simulink model "RiceCooker"  (R2023b)
settings: Solver=FixedStepAuto  StartTime=0.0  StopTime=10*60  RelTol=1e-3
undefined symbols (not defined in the file): m_0, T_0
settings Model: Creator=20181234  LastModifiedBy=20181234

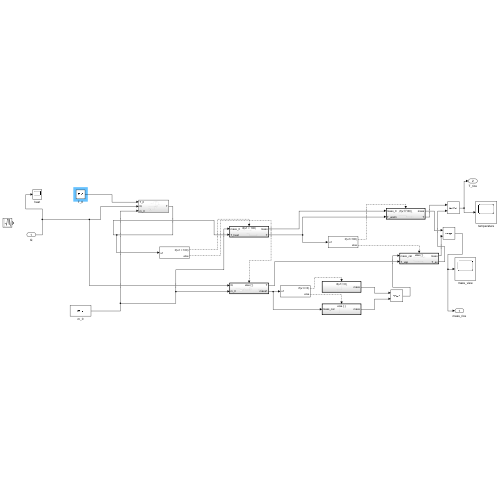
[thumbnail: Simulink's stored preview of the top-level diagram]
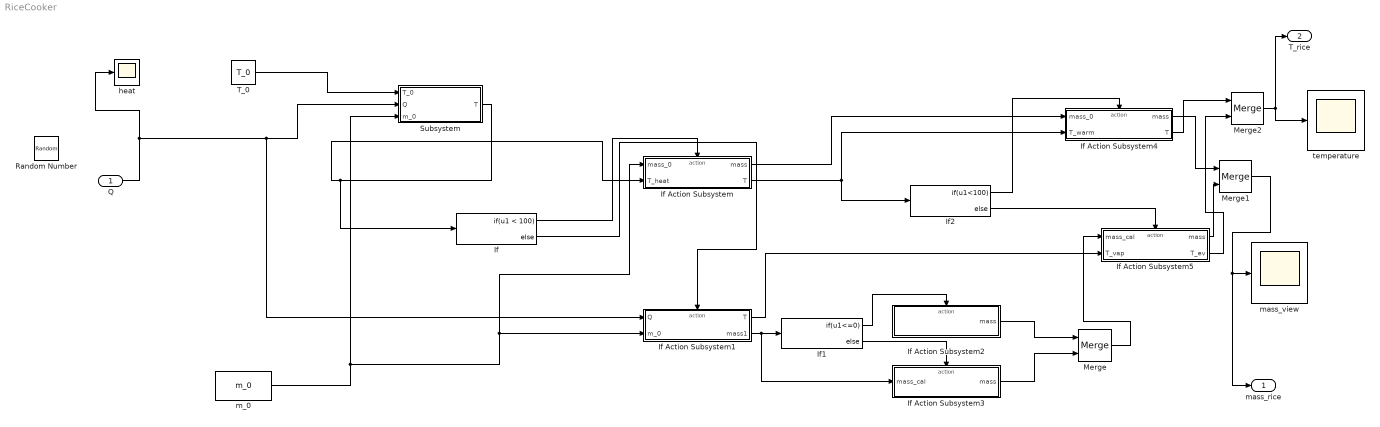
== system RiceCooker ==
  Q : Inport
  If : If  IfExpression=u1 < 100
  If Action Subsystem : Subsystem  TreatAsAtomicUnit=on
  If Action Subsystem1 : Subsystem  TreatAsAtomicUnit=on
  If Action Subsystem2 : Subsystem  TreatAsAtomicUnit=on
  If Action Subsystem3 : Subsystem  TreatAsAtomicUnit=on
  If Action Subsystem4 : Subsystem  TreatAsAtomicUnit=on
  If Action Subsystem5 : Subsystem  TreatAsAtomicUnit=on
  If1 : If  IfExpression=u1<=0
  If2 : If  IfExpression=u1<100
  Merge : Merge
  Merge1 : Merge
  Merge2 : Merge
  Random Number : RandomNumber  Mean=4500  Variance=500  Seed=65981  SampleTime=0.5
  Subsystem : Subsystem
  T_0 : Constant  Value=T_0
  heat : Scope
  m_0 : Constant  Value=m_0
  mass_view : Scope
  temperature : Scope
  mass_rice : Outport
  T_rice : Outport  Port=2
  wires:
  T_0/1 -> Subsystem/1(T_0)
  Q/1 -> heat/1, If Action Subsystem1/1(Q), Subsystem/2(Q)
  m_0/1 -> If Action Subsystem1/2(m_0), If Action Subsystem/1(mass_0), Subsystem/3(m_0)
  Subsystem/1(T) -> If/1, If Action Subsystem/2(T_heat)
  If/1 -> If Action Subsystem/Action
  If/2 -> If Action Subsystem1/Action
  If Action Subsystem/2(T) -> If Action Subsystem4/2(T_warm), If2/1
  If Action Subsystem1/2(mass1) -> If Action Subsystem3/1(mass_cal), If1/1
  If1/1 -> If Action Subsystem2/Action
  If1/2 -> If Action Subsystem3/Action
  If Action Subsystem2/1(mass) -> Merge/1
  If Action Subsystem3/1(mass) -> Merge/2
  Merge/1 -> If Action Subsystem5/1(mass_cal)
  If2/2 -> If Action Subsystem5/Action
  If2/1 -> If Action Subsystem4/Action
  If Action Subsystem4/1(mass) -> Merge1/1
  If Action Subsystem5/1(mass) -> Merge1/2
  Merge1/1 -> mass_rice/1, mass_view/1
  If Action Subsystem/1(mass) -> If Action Subsystem4/1(mass_0)
  If Action Subsystem4/2(T) -> Merge2/1
  If Action Subsystem5/2(T_ev) -> Merge2/2
  Merge2/1 -> T_rice/1, temperature/1
  If Action Subsystem1/1(T) -> If Action Subsystem5/2(T_vap)

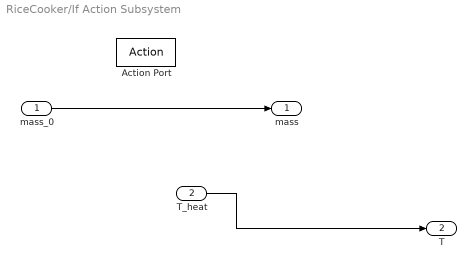
== system RiceCooker/If Action Subsystem ==
  mass_0 : Inport
  T_heat : Inport  Port=2
  Action Port : ActionPort  ActionPortLabel=if(u1 < 100)
  mass : Outport
  T : Outport  Port=2
  wires:
  mass_0/1 -> mass/1
  T_heat/1 -> T/1

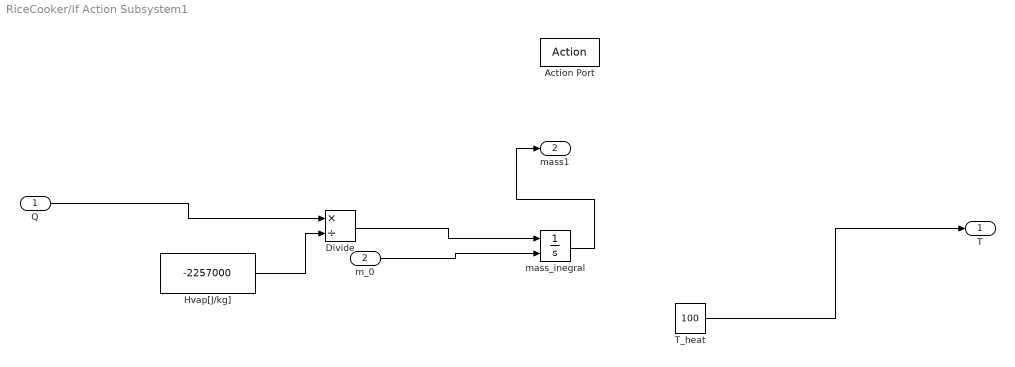
== system RiceCooker/If Action Subsystem1 ==
  Q : Inport
  m_0 : Inport  Port=2
  Action Port : ActionPort  ActionPortLabel=else
  Divide : Product  Inputs=*/
  Hvap[J/kg] : Constant  Value=-2257000
  T_heat : Constant  Value=100
  mass_inegral : Integrator  InitialConditionSource=external
  T : Outport
  mass1 : Outport  Port=2
  wires:
  Hvap[J/kg]/1 -> Divide/2
  m_0/1 -> mass_inegral/2
  mass_inegral/1 -> mass1/1
  Q/1 -> Divide/1
  Divide/1 -> mass_inegral/1
  T_heat/1 -> T/1

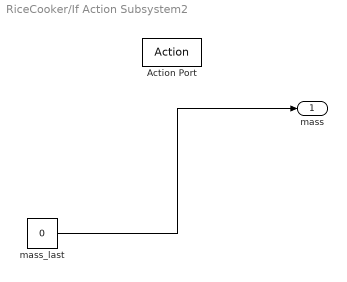
== system RiceCooker/If Action Subsystem2 ==
  Action Port : ActionPort  ActionPortLabel=if(u1<=0)
  mass_last : Constant  Value=0
  mass : Outport
  wires:
  mass_last/1 -> mass/1

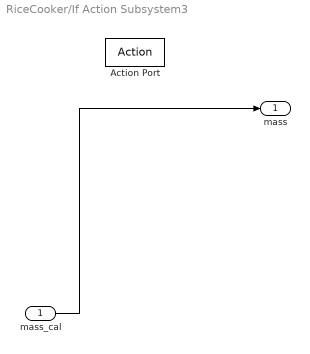
== system RiceCooker/If Action Subsystem3 ==
  mass_cal : Inport
  Action Port : ActionPort  ActionPortLabel=else
  mass : Outport
  wires:
  mass_cal/1 -> mass/1

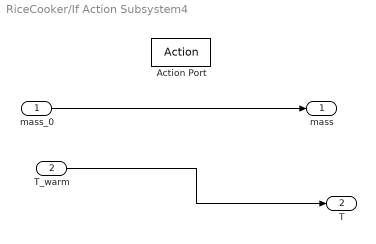
== system RiceCooker/If Action Subsystem4 ==
  mass_0 : Inport
  T_warm : Inport  Port=2
  Action Port : ActionPort  ActionPortLabel=if(u1<100)
  mass : Outport
  T : Outport  Port=2
  wires:
  mass_0/1 -> mass/1
  T_warm/1 -> T/1

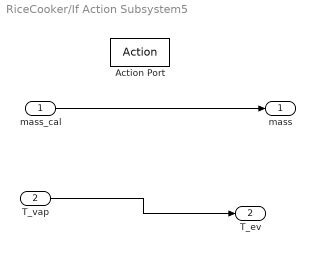
== system RiceCooker/If Action Subsystem5 ==
  mass_cal : Inport
  T_vap : Inport  Port=2
  Action Port : ActionPort  ActionPortLabel=else
  mass : Outport
  T_ev : Outport  Port=2
  wires:
  mass_cal/1 -> mass/1
  T_vap/1 -> T_ev/1

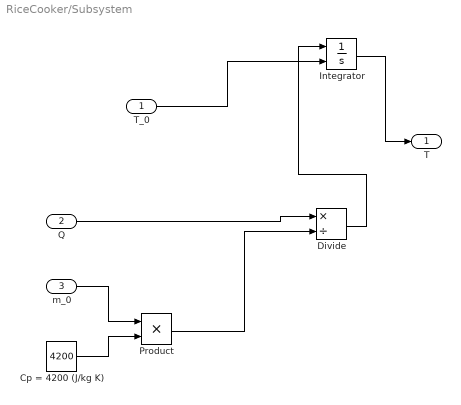
== system RiceCooker/Subsystem ==
  T_0 : Inport
  Q : Inport  Port=2
  m_0 : Inport  Port=3
  Cp = 4200 (J/kg K) : Constant  Value=4200
  Divide : Product  Inputs=*/
  Integrator : Integrator  InitialConditionSource=external
  Product : Product
  T : Outport
  wires:
  m_0/1 -> Product/1
  Divide/1 -> Integrator/1
  Cp = 4200 (J/kg K)/1 -> Product/2
  Product/1 -> Divide/2
  Integrator/1 -> T/1
  Q/1 -> Divide/1
  T_0/1 -> Integrator/2
